simulink model "db4_1"  (R2018a)
settings: Solver=ode23  StartTime=0.0  StopTime=0.5  RelTol=1e-7  AbsTol=1e-9
values from neighbouring files (symbols this model uses):
  Iaref = str2num(get(findobj('Tag','variable1'),'String'))    [simulaciones.m]
  Kpi = str2num(get(findobj('Tag','variable3'),'String'))    [graficas_a.m]    (also in graficas_b.m; simulaciones.m = Kpr*str2num(get(findobj('Tag','variable3'),'String')))
  Kpr = 20    [set_motor.m]    (also in simulaciones.m)
  Kti = 1    [set_motor.m]    (also in simulaciones.m)
  Ra = 1.2    [set_motor.m]
  Tfi = 8e-3    (= 0.008)    [set_motor.m]    (also in simulaciones.m)
  TIi = str2num(get(findobj('Tag','variable4'),'String'))    [graficas_a.m]    (also in simulaciones.m = Ta)
  Tsigma = 0.013    [set_motor.m]    (also in simulaciones.m)
settings Model: ExtModeTrigMode=oneshot  ExtModeArmWhenConnect=off  Creator=matia  LastModifiedBy=Matias
settings SolverCC: AutoScaleAbsTol=off
settings DataIOCC: SaveFormat=Array  SignalLoggingSaveFormat=ModelDataLogs  Refine=5
settings OptimizationCC: BlockReduction=off  BooleanDataType=off  LifeSpan=inf
settings DebuggingCC: SaveWithParameterizedLinksMsg=none  UnderspecifiedInitializationDetection=Classic  MergeDetectMultiDrivingBlocksExec=none  SignalResolutionControl=TryResolveAllWithWarning  MultiTaskDSMMsg=warning  MultiTaskCondExecSysMsg=none  StateNameClashWarn=warning  SFUnexpectedBacktrackingDiag=warning  SFNoUnconditionalDefaultTransitionDiag=warning  SFExecutionAtInitializationDiag=none
settings HardwareCC: ProdBitPerPointer=32  ProdBitPerSizeT=32  ProdBitPerPtrDiffT=32  ProdLargestAtomicFloat=None  ProdIntDivRoundTo=Undefined  ProdEndianess=Unspecified  ProdWordSize=32  ProdHWDeviceType=32-bit Generic  TargetUnknown=on
settings ModelReferenceCC: PropagateSignalLabelsOutOfModel=off
settings RTWCC: TemplateMakefile=grt_vc.tmf
settings CodeAppCC: StateflowObjectComments=on
settings GRTTargetCC: TargetLangStandard=C89/C90 (ANSI)  GeneratePreprocessorConditionals=Disable all  CombineOutputUpdateFcns=off  GRTInterface=on
settings ConfigComp: CovMetricSettings=dw  CovHtmlReporting=on  CovSaveCumulativeToWorkspaceVar=on  CovSaveSingleToWorkspaceVar=on  CovExternalEMLEnable=off

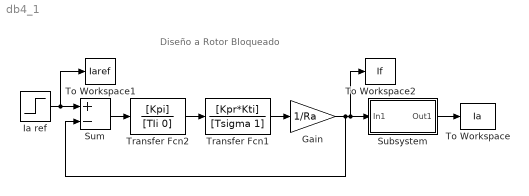
== system db4_1 ==
  note: Diseño a Rotor Bloqueado
  Gain : Gain  Gain=1/Ra  SaturateOnIntegerOverflow=on  OutDataTypeStr=Inherit: Same as input  ParamDataTypeStr=Inherit: Same as input
  "Ia ref " : Step  Time=0  After=Iaref  SampleTime=0
  Subsystem : Subsystem  mask{Tfi=Tfi, Kti=Kti}
      mask Display: disp(' (1+Tfi.s)/Kti')
  Sum : Sum  Inputs=+-  SaturateOnIntegerOverflow=on  InputSameDT=on  OutDataTypeStr=Inherit: Same as first input
  To Workspace : ToWorkspace  VariableName=Ia  SampleTime=-1
  To Workspace1 : ToWorkspace  VariableName=Iaref
  To Workspace2 : ToWorkspace  VariableName=If  SampleTime=-1
  Transfer Fcn1 : TransferFcn  Numerator=[Kpr*Kti]  Denominator=[Tsigma 1]
  Transfer Fcn2 : TransferFcn  Numerator=[Kpi]  Denominator=[TIi 0]
  wires:
  "Ia ref "/1 -> To Workspace1/1, Sum/1
  Subsystem/1(Out1) -> To Workspace/1
  Sum/1 -> Transfer Fcn2/1
  Transfer Fcn2/1 -> Transfer Fcn1/1
  Transfer Fcn1/1 -> Gain/1
  Gain/1 -> To Workspace2/1, Subsystem/1(In1), Sum/2

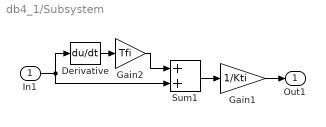
== system db4_1/Subsystem ==
  In1 : Inport
  Derivative : Derivative
  Gain1 : Gain  Gain=1/Kti  SaturateOnIntegerOverflow=on  OutDataTypeStr=Inherit: Same as input  ParamDataTypeStr=Inherit: Same as input
  Gain2 : Gain  Gain=Tfi  SaturateOnIntegerOverflow=on  OutDataTypeStr=Inherit: Same as input  ParamDataTypeStr=Inherit: Same as input
  Sum1 : Sum  SaturateOnIntegerOverflow=on  InputSameDT=on  OutDataTypeStr=Inherit: Same as first input
  Out1 : Outport
  wires:
  In1/1 -> Derivative/1, Sum1/2
  Sum1/1 -> Gain1/1
  Gain1/1 -> Out1/1
  Derivative/1 -> Gain2/1
  Gain2/1 -> Sum1/1
